simulink model "distmodel_v5"  (R2020b)
settings: Solver=FixedStepAuto  StartTime=0.0  StopTime=t_sim  FixedStep=TimeStep  RelTol=1e-3
values from neighbouring files (symbols this model uses):
  alt = 300    [main_disturbances.m]    (also in simple_propagator.m)
  c = 299792458    [main_disturbances.m]
  Cd = 2.4    [SNAP_aero_CreateTorqueProfile.m]    (also in main_disturbances.m; testsaeroSNAPmod.m)
  D = [x_th-x_cog;y_th-y_cog;z_th-z_cog]/1e3    [momentumstorage.m]
  date_IGRF = [date.year,date.month,date.day]    [main_disturbances.m]
  F_s = 1367    [main_disturbances.m]
  inc = rad2deg(inc)    [main_disturbances.m]    (also in simple_propagator.m)
  nmax = 2    [main_disturbances.m]
  nu = rad2deg(nu)    [main_disturbances.m]    (also in simple_propagator.m)
  q = 0.6    [main_disturbances.m]
  RAAN = rad2deg(RAAN)    [main_disturbances.m]    (also in simple_propagator.m)
  Use_IGRF = 0    [main_disturbances.m]
  w = find(volume(:,y,z) == 1)    [calc_torque_v1.m]    (also in main_disturbances.m = rad2deg(w); simple_propagator.m = rad2deg(w))
undefined symbols (not defined in the file or in its folder): date, DipoleMod, ecc, IonSataero, km, s, sat
libraries: vrlib x12, dspmathops x10, sharedtransform x8, aerolibutil x5, simulink_extras x4, sharedutil x2, aerolibconvert2 x1, aerolibatmos2 x1, aerolibobsolete x1, aerolibcelestial x1
(part 2 of 2)

== matlab function distmodel_v5/Time propagator/MATLAB Function ==
  data: t input; Y output; DOY output; S output
function [Y, DOY, S] = DOY(t)
Y = 2022 + fix(t/31557600);
DOY = 1+fix((t-floor(t/31557600)*31557600)/86400);
S = t - fix(t/31557600)*31557600 - (DOY-1)*86400;
